simulink model "model"  (R2014a)
(part 2 of 2)

  _CN_199309340_110000_CN_171608231_110000/RConn2 -- T_171608231__RTP/LConn2 -- _CN_34853414_110000_CN_171608231_110000/LConn2
  _CN_199309340_110000_CN_171608231_110000/RConn3 -- T_171608231__RTP/LConn3 -- _CN_34853414_110000_CN_171608231_110000/LConn3 -- bus2/LConn1
  _CN_199309340_110000_CN_129377014_110000/RConn1 -- T_129377014__HE_Vuhred/LConn1 -- _CN_198773974_110000_CN_129377014_110000/LConn1 -- _CN_34853414_110000_CN_129377014_110000/LConn1
  _CN_199309340_110000_CN_129377014_110000/RConn2 -- T_129377014__HE_Vuhred/LConn2 -- _CN_198773974_110000_CN_129377014_110000/LConn2 -- _CN_34853414_110000_CN_129377014_110000/LConn2
  _CN_199309340_110000_CN_129377014_110000/RConn3 -- T_129377014__HE_Vuhred/LConn3 -- _CN_198773974_110000_CN_129377014_110000/LConn3 -- bus3/LConn1 -- _CN_34853414_110000_CN_129377014_110000/LConn3
  _CN_121547295_110000_CN_306834171_110000/LConn1 -- T_121547295_110000_HE_Mavčiče/LConn1 -- _CN_121547295_110000_CN_35041274_110000/LConn1 -- _CN_121547295_110000_CN_167068843_110000/LConn1
  _CN_121547295_110000_CN_306834171_110000/LConn2 -- T_121547295_110000_HE_Mavčiče/LConn2 -- _CN_121547295_110000_CN_35041274_110000/LConn2 -- _CN_121547295_110000_CN_167068843_110000/LConn2
  _CN_121547295_110000_CN_306834171_110000/LConn3 -- T_121547295_110000_HE_Mavčiče/LConn3 -- _CN_121547295_110000_CN_35041274_110000/LConn3 -- _CN_121547295_110000_CN_167068843_110000/LConn3 -- bus4/LConn1
  _CN_121547295_110000_CN_306834171_110000/RConn1 -- T_306834171__RTP_Labore/LConn1 -- _CN_306834171_110000_CN_306834179_110000/LConn1
  _CN_121547295_110000_CN_306834171_110000/RConn2 -- T_306834171__RTP_Labore/LConn2 -- _CN_306834171_110000_CN_306834179_110000/LConn2
  _CN_121547295_110000_CN_306834171_110000/RConn3 -- T_306834171__RTP_Labore/LConn3 -- _CN_306834171_110000_CN_306834179_110000/LConn3 -- bus5/LConn1
  _CN_121547295_110000_CN_35041274_110000/RConn1 -- T_35041274__RTP_Okroglo/RConn1 -- _CN_306834179_110000_CN_35041274_110000/LConn1 -- L_35041274/LConn1 -- _CN_167068843_110000_CN_35041274_110000/LConn1
  _CN_121547295_110000_CN_35041274_110000/RConn2 -- T_35041274__RTP_Okroglo/RConn2 -- _CN_306834179_110000_CN_35041274_110000/LConn2 -- L_35041274/LConn2 -- _CN_167068843_110000_CN_35041274_110000/LConn2
  _CN_121547295_110000_CN_35041274_110000/RConn3 -- T_35041274__RTP_Okroglo/RConn3 -- _CN_306834179_110000_CN_35041274_110000/LConn3 -- L_35041274/LConn3 -- bus6/LConn1 -- _CN_167068843_110000_CN_35041274_110000/LConn3
  _CN_121547295_110000_CN_167068843_110000/RConn1 -- T_167068843_220000;110000_RTP_Kleče/LConn1 -- _CN_167068843_110000_CN_198965564_110000/LConn1 -- 2x110_kV_TE_TOL___Črnuče___Kleče_CN_167068843_110000_CN_186330420_110000/LConn1 -- 2x110_kV_TE_TOL___Črnuče___Kleče_CN_167068843_110000_CN_35073279_110000/LConn1 -- _CN_167068843_110000_CN_138362793_110000/LConn1 -- _CN_199456347_110000_CN_167068843_110000/LConn1 -- _CN_199456348_110000_CN_167068843_110000/LConn1 -- _CN_199131958_110000_CN_167068843_110000/LConn1 -- _CN_167068843_110000_CN_306834196_110000/LConn1 -- _CN_167068843_110000_CN_35041274_110000/RConn1
  _CN_121547295_110000_CN_167068843_110000/RConn2 -- T_167068843_220000;110000_RTP_Kleče/LConn2 -- _CN_167068843_110000_CN_198965564_110000/LConn2 -- 2x110_kV_TE_TOL___Črnuče___Kleče_CN_167068843_110000_CN_186330420_110000/LConn2 -- 2x110_kV_TE_TOL___Črnuče___Kleče_CN_167068843_110000_CN_35073279_110000/LConn2 -- _CN_167068843_110000_CN_138362793_110000/LConn2 -- _CN_199456347_110000_CN_167068843_110000/LConn2 -- _CN_199456348_110000_CN_167068843_110000/LConn2 -- _CN_199131958_110000_CN_167068843_110000/LConn2 -- _CN_167068843_110000_CN_306834196_110000/LConn2 -- _CN_167068843_110000_CN_35041274_110000/RConn2
  _CN_121547295_110000_CN_167068843_110000/RConn3 -- T_167068843_220000;110000_RTP_Kleče/LConn3 -- _CN_167068843_110000_CN_198965564_110000/LConn3 -- 2x110_kV_TE_TOL___Črnuče___Kleče_CN_167068843_110000_CN_186330420_110000/LConn3 -- 2x110_kV_TE_TOL___Črnuče___Kleče_CN_167068843_110000_CN_35073279_110000/LConn3 -- _CN_167068843_110000_CN_138362793_110000/LConn3 -- bus7/LConn1 -- _CN_199456347_110000_CN_167068843_110000/LConn3 -- _CN_199456348_110000_CN_167068843_110000/LConn3 -- _CN_199131958_110000_CN_167068843_110000/LConn3 -- _CN_167068843_110000_CN_306834196_110000/LConn3 -- _CN_167068843_110000_CN_35041274_110000/RConn3
  _CN_34853414_110000_CN_171608231_110000/RConn1 -- T_34853414__RTP_Pekre/LConn1 -- _CN_34853414_110000_CN_129377014_110000/RConn1 -- _CN_34853414_110000_CN_113578863_110000/LConn1 -- _CN_34853414_110000_CN_171257375_110000/LConn1 -- _CN_34853414_110000_CN_171247394_110000/LConn1 -- 110kV_podzemni_kabel_RTP_Koroška_vrata_RTP_Pekre_CN_34853414_110000_CN_171242382_110000/LConn1 -- _CN_34853414_110000_CN_170856590_110000/LConn1
  _CN_34853414_110000_CN_171608231_110000/RConn2 -- T_34853414__RTP_Pekre/LConn2 -- _CN_34853414_110000_CN_129377014_110000/RConn2 -- _CN_34853414_110000_CN_113578863_110000/LConn2 -- _CN_34853414_110000_CN_171257375_110000/LConn2 -- _CN_34853414_110000_CN_171247394_110000/LConn2 -- 110kV_podzemni_kabel_RTP_Koroška_vrata_RTP_Pekre_CN_34853414_110000_CN_171242382_110000/LConn2 -- _CN_34853414_110000_CN_170856590_110000/LConn2
  _CN_34853414_110000_CN_171608231_110000/RConn3 -- T_34853414__RTP_Pekre/LConn3 -- _CN_34853414_110000_CN_129377014_110000/RConn3 -- bus8/LConn1 -- _CN_34853414_110000_CN_113578863_110000/LConn3 -- _CN_34853414_110000_CN_171257375_110000/LConn3 -- _CN_34853414_110000_CN_171247394_110000/LConn3 -- 110kV_podzemni_kabel_RTP_Koroška_vrata_RTP_Pekre_CN_34853414_110000_CN_171242382_110000/LConn3 -- _CN_34853414_110000_CN_170856590_110000/LConn3
  _CN_34853414_110000_CN_113578863_110000/RConn1 -- T_113578863__RTP_Maribor/RConn1 -- 110kV_RTP_Maribor_RTP_Lenart_CN_113578863_110000_CN_171246987_110000/LConn1 -- 110_kV_RTP_Maribor_RTP_Melje_CN_113578863_110000_CN_171242383_110000/LConn1 -- L_113578863/LConn1 -- 110kV_RTP_Maribor_RTP_Cirkovce_CN_113568896_110000_CN_113578863_110000/LConn1
  _CN_34853414_110000_CN_113578863_110000/RConn2 -- T_113578863__RTP_Maribor/RConn2 -- 110kV_RTP_Maribor_RTP_Lenart_CN_113578863_110000_CN_171246987_110000/LConn2 -- 110_kV_RTP_Maribor_RTP_Melje_CN_113578863_110000_CN_171242383_110000/LConn2 -- L_113578863/LConn2 -- 110kV_RTP_Maribor_RTP_Cirkovce_CN_113568896_110000_CN_113578863_110000/LConn2
  _CN_34853414_110000_CN_113578863_110000/RConn3 -- T_113578863__RTP_Maribor/RConn3 -- 110kV_RTP_Maribor_RTP_Lenart_CN_113578863_110000_CN_171246987_110000/LConn3 -- 110_kV_RTP_Maribor_RTP_Melje_CN_113578863_110000_CN_171242383_110000/LConn3 -- L_113578863/LConn3 -- bus9/LConn1 -- 110kV_RTP_Maribor_RTP_Cirkovce_CN_113568896_110000_CN_113578863_110000/LConn3
  T_171257375__RTP_Slovenska_BIstrica/LConn1 -- _CN_34853414_110000_CN_171257375_110000/RConn1
  T_171257375__RTP_Slovenska_BIstrica/LConn2 -- _CN_34853414_110000_CN_171257375_110000/RConn2
  _CN_34853414_110000_CN_171257375_110000/RConn3 -- T_171257375__RTP_Slovenska_BIstrica/LConn3 -- bus10/LConn1
  T_171247394__HE_Mariborski_otok/LConn1 -- _CN_34853414_110000_CN_171247394_110000/RConn1
  T_171247394__HE_Mariborski_otok/LConn2 -- _CN_34853414_110000_CN_171247394_110000/RConn2
  _CN_34853414_110000_CN_171247394_110000/RConn3 -- T_171247394__HE_Mariborski_otok/LConn3 -- bus11/LConn1
  110kV_podzemni_kabel_RTP_Koroška_vrata_RTP_Pekre_CN_34853414_110000_CN_171242382_110000/RConn1 -- T_171242382__RTP_Koroška_vrata/LConn1 -- 110kV_podvodni_kabel_RTP_Koroška_vrata__RTP_Melje_CN_171242382_110000_CN_171242383_110000/LConn1
  110kV_podzemni_kabel_RTP_Koroška_vrata_RTP_Pekre_CN_34853414_110000_CN_171242382_110000/RConn2 -- T_171242382__RTP_Koroška_vrata/LConn2 -- 110kV_podvodni_kabel_RTP_Koroška_vrata__RTP_Melje_CN_171242382_110000_CN_171242383_110000/LConn2
  110kV_podzemni_kabel_RTP_Koroška_vrata_RTP_Pekre_CN_34853414_110000_CN_171242382_110000/RConn3 -- T_171242382__RTP_Koroška_vrata/LConn3 -- 110kV_podvodni_kabel_RTP_Koroška_vrata__RTP_Melje_CN_171242382_110000_CN_171242383_110000/LConn3 -- bus12/LConn1
  T_170856590__RTP_Dobrava/LConn1 -- _CN_34853414_110000_CN_170856590_110000/RConn1
  T_170856590__RTP_Dobrava/LConn2 -- _CN_34853414_110000_CN_170856590_110000/RConn2
  _CN_34853414_110000_CN_170856590_110000/RConn3 -- T_170856590__RTP_Dobrava/LConn3 -- bus13/LConn1
  T_280821359__/LConn1 -- _CN_280821359_110000_CN_171277752_110000/LConn1
  T_280821359__/LConn2 -- _CN_280821359_110000_CN_171277752_110000/LConn2
  _CN_280821359_110000_CN_171277752_110000/LConn3 -- T_280821359__/LConn3 -- bus14/LConn1
  T_171277752__RTP_Slovenske_Konjice/LConn1 -- _CN_280821359_110000_CN_171277752_110000/RConn1
  T_171277752__RTP_Slovenske_Konjice/LConn2 -- _CN_280821359_110000_CN_171277752_110000/RConn2
  _CN_280821359_110000_CN_171277752_110000/RConn3 -- T_171277752__RTP_Slovenske_Konjice/LConn3 -- bus15/LConn1
  _CN_171047486_110000_CN_113568896_110000/LConn1 -- T_171047486__RTP_Kidričevo/LConn1 -- _CN_171047486_110000_CN_171223453_110000/LConn1 -- _CN_171047486_110000_CN_171127243_110000/LConn1
  _CN_171047486_110000_CN_113568896_110000/LConn2 -- T_171047486__RTP_Kidričevo/LConn2 -- _CN_171047486_110000_CN_171223453_110000/LConn2 -- _CN_171047486_110000_CN_171127243_110000/LConn2
  _CN_171047486_110000_CN_113568896_110000/LConn3 -- T_171047486__RTP_Kidričevo/LConn3 -- _CN_171047486_110000_CN_171223453_110000/LConn3 -- _CN_171047486_110000_CN_171127243_110000/LConn3 -- bus16/LConn1
  _CN_171047486_110000_CN_113568896_110000/RConn1 -- T_113568896__RTP_Cirkovce/LConn1 -- _CN_280821361_110000_CN_113568896_110000/LConn1 -- 110kV_RTP_Maribor_RTP_Cirkovce_CN_113568896_110000_CN_113578863_110000/RConn1 -- _CN_113568896_110000_CN_170978399_110000/LConn1
  _CN_171047486_110000_CN_113568896_110000/RConn2 -- T_113568896__RTP_Cirkovce/LConn2 -- _CN_280821361_110000_CN_113568896_110000/LConn2 -- 110kV_RTP_Maribor_RTP_Cirkovce_CN_113568896_110000_CN_113578863_110000/RConn2 -- _CN_113568896_110000_CN_170978399_110000/LConn2
  _CN_171047486_110000_CN_113568896_110000/RConn3 -- T_113568896__RTP_Cirkovce/LConn3 -- _CN_280821361_110000_CN_113568896_110000/LConn3 -- 110kV_RTP_Maribor_RTP_Cirkovce_CN_113568896_110000_CN_113578863_110000/RConn3 -- _CN_113568896_110000_CN_170978399_110000/LConn3 -- bus17/LConn1
  _CN_171047486_110000_CN_171223453_110000/RConn1 -- G_171223453_HE_Formin/RConn1 -- _CN_171229302_110000_CN_171223453_110000/LConn1 -- _CN_280821361_110000_CN_171223453_110000/LConn1
  _CN_171047486_110000_CN_171223453_110000/RConn2 -- G_171223453_HE_Formin/RConn2 -- _CN_171229302_110000_CN_171223453_110000/LConn2 -- _CN_280821361_110000_CN_171223453_110000/LConn2
  _CN_171047486_110000_CN_171223453_110000/RConn3 -- G_171223453_HE_Formin/RConn3 -- _CN_171229302_110000_CN_171223453_110000/LConn3 -- bus18/LConn1 -- _CN_280821361_110000_CN_171223453_110000/LConn3
  T_171127243__RTP_Ptuj/LConn1 -- _CN_171047486_110000_CN_171127243_110000/RConn1
  T_171127243__RTP_Ptuj/LConn2 -- _CN_171047486_110000_CN_171127243_110000/RConn2
  _CN_171047486_110000_CN_171127243_110000/RConn3 -- T_171127243__RTP_Ptuj/LConn3 -- bus19/LConn1
  T_198587974__RTP/LConn1 -- Podlog_Mozirje_CN_198587974_110000_CN_119244495_110000/LConn1
  T_198587974__RTP/LConn2 -- Podlog_Mozirje_CN_198587974_110000_CN_119244495_110000/LConn2
  Podlog_Mozirje_CN_198587974_110000_CN_119244495_110000/LConn3 -- T_198587974__RTP/LConn3 -- bus20/LConn1
  Podlog_Mozirje_CN_198587974_110000_CN_119244495_110000/RConn1 -- T_119244495__RTP_Podlog/RConn1 -- _CN_280821368_110000_CN_119244495_110000/LConn1 -- L_119244495/LConn1
  Podlog_Mozirje_CN_198587974_110000_CN_119244495_110000/RConn2 -- T_119244495__RTP_Podlog/RConn2 -- _CN_280821368_110000_CN_119244495_110000/LConn2 -- L_119244495/LConn2
  Podlog_Mozirje_CN_198587974_110000_CN_119244495_110000/RConn3 -- T_119244495__RTP_Podlog/RConn3 -- _CN_280821368_110000_CN_119244495_110000/LConn3 -- L_119244495/LConn3 -- bus21/LConn1
  T_199456336__RTP_Bršljin/LConn1 -- _CN_199456336_110000_CN_198740080_110000/LConn1
  T_199456336__RTP_Bršljin/LConn2 -- _CN_199456336_110000_CN_198740080_110000/LConn2
  _CN_199456336_110000_CN_198740080_110000/LConn3 -- T_199456336__RTP_Bršljin/LConn3 -- bus22/LConn1
  _CN_199456336_110000_CN_198740080_110000/RConn1 -- T_198740080_110000_RP_Hudo/LConn1 -- _CN_198740080_110000_CN_262103358_110000/LConn1 -- _CN_198740080_110000_CN_262103381_110000/LConn1
  _CN_199456336_110000_CN_198740080_110000/RConn2 -- T_198740080_110000_RP_Hudo/LConn2 -- _CN_198740080_110000_CN_262103358_110000/LConn2 -- _CN_198740080_110000_CN_262103381_110000/LConn2
  _CN_199456336_110000_CN_198740080_110000/RConn3 -- T_198740080_110000_RP_Hudo/LConn3 -- _CN_198740080_110000_CN_262103358_110000/LConn3 -- _CN_198740080_110000_CN_262103381_110000/LConn3 -- bus23/LConn1
  T_199456340_110000_RTP_Grosuplje/LConn1 -- _CN_199456340_110000_CN_138362793_110000/LConn1
  T_199456340_110000_RTP_Grosuplje/LConn2 -- _CN_199456340_110000_CN_138362793_110000/LConn2
  _CN_199456340_110000_CN_138362793_110000/LConn3 -- T_199456340_110000_RTP_Grosuplje/LConn3 -- bus24/LConn1
  _CN_199456340_110000_CN_138362793_110000/RConn1 -- T_138362793__RTP_Beričevo/RConn1 -- _CN_167068843_110000_CN_138362793_110000/RConn1 -- 2x110_kV_TE_TOL___Polje___Beričevo_CN_138362793_110000_CN_35073279_110000/LConn1 -- L_138362793/LConn1
  _CN_199456340_110000_CN_138362793_110000/RConn2 -- T_138362793__RTP_Beričevo/RConn2 -- _CN_167068843_110000_CN_138362793_110000/RConn2 -- 2x110_kV_TE_TOL___Polje___Beričevo_CN_138362793_110000_CN_35073279_110000/LConn2 -- L_138362793/LConn2
  _CN_199456340_110000_CN_138362793_110000/RConn3 -- T_138362793__RTP_Beričevo/RConn3 -- _CN_167068843_110000_CN_138362793_110000/RConn3 -- 2x110_kV_TE_TOL___Polje___Beričevo_CN_138362793_110000_CN_35073279_110000/LConn3 -- L_138362793/LConn3 -- bus25/LConn1
  T_199456341__RTP_Kamnik/LConn1 -- Domžale___Kamnik_CN_199456341_110000_CN_198965564_110000/LConn1
  T_199456341__RTP_Kamnik/LConn2 -- Domžale___Kamnik_CN_199456341_110000_CN_198965564_110000/LConn2
  Domžale___Kamnik_CN_199456341_110000_CN_198965564_110000/LConn3 -- T_199456341__RTP_Kamnik/LConn3 -- bus26/LConn1
  Domžale___Kamnik_CN_199456341_110000_CN_198965564_110000/RConn1 -- T_198965564__RTP_Domžale/LConn1 -- _CN_167068843_110000_CN_198965564_110000/RConn1
  Domžale___Kamnik_CN_199456341_110000_CN_198965564_110000/RConn2 -- T_198965564__RTP_Domžale/LConn2 -- _CN_167068843_110000_CN_198965564_110000/RConn2
  Domžale___Kamnik_CN_199456341_110000_CN_198965564_110000/RConn3 -- T_198965564__RTP_Domžale/LConn3 -- _CN_167068843_110000_CN_198965564_110000/RConn3 -- bus27/LConn1
  T_199456345__RTP_Potoška_vas/LConn1 -- _CN_199456345_110000_CN_286599451_110000/LConn1
  T_199456345__RTP_Potoška_vas/LConn2 -- _CN_199456345_110000_CN_286599451_110000/LConn2
  _CN_199456345_110000_CN_286599451_110000/LConn3 -- T_199456345__RTP_Potoška_vas/LConn3 -- bus28/LConn1
  T_286599451__RTP_Trbovlje/LConn1 -- _CN_199456345_110000_CN_286599451_110000/RConn1
  T_286599451__RTP_Trbovlje/LConn2 -- _CN_199456345_110000_CN_286599451_110000/RConn2
  _CN_199456345_110000_CN_286599451_110000/RConn3 -- T_286599451__RTP_Trbovlje/LConn3 -- bus29/LConn1
  T_199456347__RTP_Vič/LConn1 -- _CN_199456347_110000_CN_167068843_110000/RConn1
  T_199456347__RTP_Vič/LConn2 -- _CN_199456347_110000_CN_167068843_110000/RConn2
  _CN_199456347_110000_CN_167068843_110000/RConn3 -- T_199456347__RTP_Vič/LConn3 -- bus30/LConn1
  T_199456348__RTP_Šiška/LConn1 -- _CN_199456348_110000_CN_167068843_110000/RConn1
  T_199456348__RTP_Šiška/LConn2 -- _CN_199456348_110000_CN_167068843_110000/RConn2
  _CN_199456348_110000_CN_167068843_110000/RConn3 -- T_199456348__RTP_Šiška/LConn3 -- bus31/LConn1
  T_198740079__/LConn1 -- _CN_198740079_110000_CN_262103381_110000/LConn1
  T_198740079__/LConn2 -- _CN_198740079_110000_CN_262103381_110000/LConn2
  _CN_198740079_110000_CN_262103381_110000/LConn3 -- T_198740079__/LConn3 -- bus32/LConn1
  _CN_198740079_110000_CN_262103381_110000/RConn1 -- T_262103381__/LConn1 -- _CN_198740080_110000_CN_262103381_110000/RConn1
  _CN_198740079_110000_CN_262103381_110000/RConn2 -- T_262103381__/LConn2 -- _CN_198740080_110000_CN_262103381_110000/RConn2
  _CN_198740079_110000_CN_262103381_110000/RConn3 -- T_262103381__/LConn3 -- _CN_198740080_110000_CN_262103381_110000/RConn3 -- bus33/LConn1
  _CN_306794096_110000_CN_370156011_110000/LConn1 -- T_306794096_110000_HE_Plave/LConn1 -- _CN_306794096_110000_CN_369889751_110000/LConn1
  _CN_306794096_110000_CN_370156011_110000/LConn2 -- T_306794096_110000_HE_Plave/LConn2 -- _CN_306794096_110000_CN_369889751_110000/LConn2
  _CN_306794096_110000_CN_370156011_110000/LConn3 -- T_306794096_110000_HE_Plave/LConn3 -- _CN_306794096_110000_CN_369889751_110000/LConn3 -- bus34/LConn1
  T_370156011__RTP_Anhovo/LConn1 -- _CN_306794096_110000_CN_370156011_110000/RConn1
  T_370156011__RTP_Anhovo/LConn2 -- _CN_306794096_110000_CN_370156011_110000/RConn2
  _CN_306794096_110000_CN_370156011_110000/RConn3 -- T_370156011__RTP_Anhovo/LConn3 -- bus35/LConn1
  _CN_306794096_110000_CN_369889751_110000/RConn1 -- G_369889751_ČHE_Avče/RConn1 -- _CN_306692448_110000_CN_369889751_110000/LConn1
  _CN_306794096_110000_CN_369889751_110000/RConn2 -- G_369889751_ČHE_Avče/RConn2 -- _CN_306692448_110000_CN_369889751_110000/LConn2
  _CN_306794096_110000_CN_369889751_110000/RConn3 -- G_369889751_ČHE_Avče/RConn3 -- _CN_306692448_110000_CN_369889751_110000/LConn3 -- bus36/LConn1
  _CN_280821361_110000_CN_280821367_110000/LConn1 -- T_280821361__/LConn1 -- _CN_280821361_110000_CN_171223453_110000/RConn1 -- _CN_280821361_110000_CN_113568896_110000/RConn1
  _CN_280821361_110000_CN_280821367_110000/LConn2 -- T_280821361__/LConn2 -- _CN_280821361_110000_CN_171223453_110000/RConn2 -- _CN_280821361_110000_CN_113568896_110000/RConn2
  _CN_280821361_110000_CN_280821367_110000/LConn3 -- T_280821361__/LConn3 -- _CN_280821361_110000_CN_171223453_110000/RConn3 -- _CN_280821361_110000_CN_113568896_110000/RConn3 -- bus37/LConn1
  T_280821367__/LConn1 -- _CN_280821361_110000_CN_280821367_110000/RConn1
  T_280821367__/LConn2 -- _CN_280821361_110000_CN_280821367_110000/RConn2
  _CN_280821361_110000_CN_280821367_110000/RConn3 -- T_280821367__/LConn3 -- bus38/LConn1
  _CN_199131958_110000_CN_167068843_110000/RConn1 -- T_199131958__RTP_Logatec/LConn1 -- _CN_199131958_110000_CN_199131955_110000/LConn1
  _CN_199131958_110000_CN_167068843_110000/RConn2 -- T_199131958__RTP_Logatec/LConn2 -- _CN_199131958_110000_CN_199131955_110000/LConn2
  _CN_199131958_110000_CN_167068843_110000/RConn3 -- T_199131958__RTP_Logatec/LConn3 -- _CN_199131958_110000_CN_199131955_110000/LConn3 -- bus39/LConn1
  T_199131955__RTP_Vrhnika/LConn1 -- _CN_199131958_110000_CN_199131955_110000/RConn1
  T_199131955__RTP_Vrhnika/LConn2 -- _CN_199131958_110000_CN_199131955_110000/RConn2
  _CN_199131958_110000_CN_199131955_110000/RConn3 -- T_199131955__RTP_Vrhnika/LConn3 -- bus40/LConn1
  T_172406389__RTP_Radenci/LConn1 -- RTP_Murska_Sobota_RTP_Radenci_CN_172406389_110000_CN_172405235_110000/LConn1
  T_172406389__RTP_Radenci/LConn2 -- RTP_Murska_Sobota_RTP_Radenci_CN_172406389_110000_CN_172405235_110000/LConn2
  RTP_Murska_Sobota_RTP_Radenci_CN_172406389_110000_CN_172405235_110000/LConn3 -- T_172406389__RTP_Radenci/LConn3 -- bus41/LConn1
  RTP_Murska_Sobota_RTP_Radenci_CN_172406389_110000_CN_172405235_110000/RConn1 -- T_172405235__RTP_Murska_Sobota/LConn1 -- RTP_Ljutomer_RTP_Murska_Sobota_CN_171229302_110000_CN_172405235_110000/LConn1
  RTP_Murska_Sobota_RTP_Radenci_CN_172406389_110000_CN_172405235_110000/RConn2 -- T_172405235__RTP_Murska_Sobota/LConn2 -- RTP_Ljutomer_RTP_Murska_Sobota_CN_171229302_110000_CN_172405235_110000/LConn2
  RTP_Murska_Sobota_RTP_Radenci_CN_172406389_110000_CN_172405235_110000/RConn3 -- T_172405235__RTP_Murska_Sobota/LConn3 -- RTP_Ljutomer_RTP_Murska_Sobota_CN_171229302_110000_CN_172405235_110000/LConn3 -- bus42/LConn1
  _CN_171229302_110000_CN_200118427_110000/LConn1 -- T_171229302__RTP_Ljutomer/LConn1 -- RTP_Ljutomer_RTP_Murska_Sobota_CN_171229302_110000_CN_172405235_110000/RConn1 -- _CN_171229302_110000_CN_171227992_110000/LConn1 -- _CN_171229302_110000_CN_171223453_110000/RConn1
  _CN_171229302_110000_CN_200118427_110000/LConn2 -- T_171229302__RTP_Ljutomer/LConn2 -- RTP_Ljutomer_RTP_Murska_Sobota_CN_171229302_110000_CN_172405235_110000/RConn2 -- _CN_171229302_110000_CN_171227992_110000/LConn2 -- _CN_171229302_110000_CN_171223453_110000/RConn2
  _CN_171229302_110000_CN_200118427_110000/LConn3 -- T_171229302__RTP_Ljutomer/LConn3 -- RTP_Ljutomer_RTP_Murska_Sobota_CN_171229302_110000_CN_172405235_110000/RConn3 -- _CN_171229302_110000_CN_171227992_110000/LConn3 -- _CN_171229302_110000_CN_171223453_110000/RConn3 -- bus43/LConn1
  T_200118427__/LConn1 -- _CN_171229302_110000_CN_200118427_110000/RConn1
  T_200118427__/LConn2 -- _CN_171229302_110000_CN_200118427_110000/RConn2
  _CN_171229302_110000_CN_200118427_110000/RConn3 -- T_200118427__/LConn3 -- bus44/LConn1
  T_171227992__RTP_Ormož/LConn1 -- _CN_171229302_110000_CN_171227992_110000/RConn1
  T_171227992__RTP_Ormož/LConn2 -- _CN_171229302_110000_CN_171227992_110000/RConn2
  _CN_171229302_110000_CN_171227992_110000/RConn3 -- T_171227992__RTP_Ormož/LConn3 -- bus45/LConn1
  T_280821368__/LConn1 -- _CN_280821368_110000_CN_119244495_110000/RConn1
  T_280821368__/LConn2 -- _CN_280821368_110000_CN_119244495_110000/RConn2
  _CN_280821368_110000_CN_119244495_110000/RConn3 -- T_280821368__/LConn3 -- bus46/LConn1
  G_170978399_HE_Zlatoličje/RConn1 -- _CN_113568896_110000_CN_170978399_110000/RConn1
  G_170978399_HE_Zlatoličje/RConn2 -- _CN_113568896_110000_CN_170978399_110000/RConn2
  _CN_113568896_110000_CN_170978399_110000/RConn3 -- G_170978399_HE_Zlatoličje/RConn3 -- bus47/LConn1
  T_262103358__/LConn1 -- _CN_198740080_110000_CN_262103358_110000/RConn1
  T_262103358__/LConn2 -- _CN_198740080_110000_CN_262103358_110000/RConn2
  _CN_198740080_110000_CN_262103358_110000/RConn3 -- T_262103358__/LConn3 -- bus48/LConn1
  DV_Krapina___Straža_CN_159593130_110000_CN_208625989_110000/LConn1 -- T_159593130__TS_Straža/LConn1 -- DV_Ivanec___Straža_CN_159593130_110000_CN_99634141_110000/LConn1
  DV_Krapina___Straža_CN_159593130_110000_CN_208625989_110000/LConn2 -- T_159593130__TS_Straža/LConn2 -- DV_Ivanec___Straža_CN_159593130_110000_CN_99634141_110000/LConn2
  DV_Krapina___Straža_CN_159593130_110000_CN_208625989_110000/LConn3 -- T_159593130__TS_Straža/LConn3 -- DV_Ivanec___Straža_CN_159593130_110000_CN_99634141_110000/LConn3 -- bus49/LConn1
  T_208625989__/LConn1 -- DV_Krapina___Straža_CN_159593130_110000_CN_208625989_110000/RConn1
  T_208625989__/LConn2 -- DV_Krapina___Straža_CN_159593130_110000_CN_208625989_110000/RConn2
  DV_Krapina___Straža_CN_159593130_110000_CN_208625989_110000/RConn3 -- T_208625989__/LConn3 -- bus50/LConn1
  T_99634141__TS_Ivanec/LConn1 -- DV_Ivanec___Straža_CN_159593130_110000_CN_99634141_110000/RConn1
  T_99634141__TS_Ivanec/LConn2 -- DV_Ivanec___Straža_CN_159593130_110000_CN_99634141_110000/RConn2
  DV_Ivanec___Straža_CN_159593130_110000_CN_99634141_110000/RConn3 -- T_99634141__TS_Ivanec/LConn3 -- bus51/LConn1
  T_306834196__RTP_Škofja_Loka/LConn1 -- _CN_167068843_110000_CN_306834196_110000/RConn1
  T_306834196__RTP_Škofja_Loka/LConn2 -- _CN_167068843_110000_CN_306834196_110000/RConn2
  _CN_167068843_110000_CN_306834196_110000/RConn3 -- T_306834196__RTP_Škofja_Loka/LConn3 -- bus52/LConn1
  T_186330420__RTP_Črnuče/LConn1 -- 2x110_kV_TE_TOL___Črnuče___Kleče_CN_167068843_110000_CN_186330420_110000/RConn1
  T_186330420__RTP_Črnuče/LConn2 -- 2x110_kV_TE_TOL___Črnuče___Kleče_CN_167068843_110000_CN_186330420_110000/RConn2
  2x110_kV_TE_TOL___Črnuče___Kleče_CN_167068843_110000_CN_186330420_110000/RConn3 -- T_186330420__RTP_Črnuče/LConn3 -- bus53/LConn1
  2x110_kV_TE_TOL___Črnuče___Kleče_CN_167068843_110000_CN_35073279_110000/RConn1 -- G_35073279_Termoelektrarna_Toplarna_Ljubljana/RConn1 -- 2x110_kV_TE_TOL___Polje___Beričevo_CN_138362793_110000_CN_35073279_110000/RConn1 -- 110_kV_TE_TOL___Polje_CN_138362817_110000_CN_35073279_110000/LConn1
  2x110_kV_TE_TOL___Črnuče___Kleče_CN_167068843_110000_CN_35073279_110000/RConn2 -- G_35073279_Termoelektrarna_Toplarna_Ljubljana/RConn2 -- 2x110_kV_TE_TOL___Polje___Beričevo_CN_138362793_110000_CN_35073279_110000/RConn2 -- 110_kV_TE_TOL___Polje_CN_138362817_110000_CN_35073279_110000/LConn2
  2x110_kV_TE_TOL___Črnuče___Kleče_CN_167068843_110000_CN_35073279_110000/RConn3 -- G_35073279_Termoelektrarna_Toplarna_Ljubljana/RConn3 -- 2x110_kV_TE_TOL___Polje___Beričevo_CN_138362793_110000_CN_35073279_110000/RConn3 -- 110_kV_TE_TOL___Polje_CN_138362817_110000_CN_35073279_110000/LConn3 -- bus54/LConn1
  T_376534710__RTP/LConn1 -- Ajdovščina___Divača_CN_376534710_110000_CN_96747435_110000/LConn1
  T_376534710__RTP/LConn2 -- Ajdovščina___Divača_CN_376534710_110000_CN_96747435_110000/LConn2
  Ajdovščina___Divača_CN_376534710_110000_CN_96747435_110000/LConn3 -- T_376534710__RTP/LConn3 -- bus55/LConn1
  Ajdovščina___Divača_CN_376534710_110000_CN_96747435_110000/RConn1 -- T_96747435_400000;220000;110000_RTP_Divača/RConn1 -- _CN_199389074_110000_CN_96747435_110000/LConn1 -- L_96747435/LConn1 -- _CN_199131954_110000_CN_96747435_110000/LConn1 -- Divača___Sežana_CN_208270146_110000_CN_96747435_110000/LConn1
  Ajdovščina___Divača_CN_376534710_110000_CN_96747435_110000/RConn2 -- T_96747435_400000;220000;110000_RTP_Divača/RConn2 -- _CN_199389074_110000_CN_96747435_110000/LConn2 -- L_96747435/LConn2 -- _CN_199131954_110000_CN_96747435_110000/LConn2 -- Divača___Sežana_CN_208270146_110000_CN_96747435_110000/LConn2
  Ajdovščina___Divača_CN_376534710_110000_CN_96747435_110000/RConn3 -- T_96747435_400000;220000;110000_RTP_Divača/RConn3 -- _CN_199389074_110000_CN_96747435_110000/LConn3 -- L_96747435/LConn3 -- bus56/LConn1 -- _CN_199131954_110000_CN_96747435_110000/LConn3 -- Divača___Sežana_CN_208270146_110000_CN_96747435_110000/LConn3
  T_132468928_110000_Kraftwerk_Koralpe/LConn1 -- Lavamünd___Koralpe_CN_132468928_110000_CN_98291700_110000/LConn1
  T_132468928_110000_Kraftwerk_Koralpe/LConn2 -- Lavamünd___Koralpe_CN_132468928_110000_CN_98291700_110000/LConn2
  Lavamünd___Koralpe_CN_132468928_110000_CN_98291700_110000/LConn3 -- T_132468928_110000_Kraftwerk_Koralpe/LConn3 -- bus57/LConn1
  G_98291700_Kraftwerk_Lavamünd/RConn1 -- Lavamünd___Koralpe_CN_132468928_110000_CN_98291700_110000/RConn1
  G_98291700_Kraftwerk_Lavamünd/RConn2 -- Lavamünd___Koralpe_CN_132468928_110000_CN_98291700_110000/RConn2
  Lavamünd___Koralpe_CN_132468928_110000_CN_98291700_110000/RConn3 -- G_98291700_Kraftwerk_Lavamünd/RConn3 -- bus58/LConn1
  T_161693379__RTP/LConn1 -- _CN_161693379_110000_CN_198773972_110000/LConn1
  T_161693379__RTP/LConn2 -- _CN_161693379_110000_CN_198773972_110000/LConn2
  _CN_161693379_110000_CN_198773972_110000/LConn3 -- T_161693379__RTP/LConn3 -- bus59/LConn1
  _CN_161693379_110000_CN_198773972_110000/RConn1 -- T_198773972__/LConn1 -- _CN_198773972_110000_CN_198773974_110000/LConn1
  _CN_161693379_110000_CN_198773972_110000/RConn2 -- T_198773972__/LConn2 -- _CN_198773972_110000_CN_198773974_110000/LConn2
  _CN_161693379_110000_CN_198773972_110000/RConn3 -- T_198773972__/LConn3 -- _CN_198773972_110000_CN_198773974_110000/LConn3 -- bus60/LConn1
  T_128572102__TS_Matulji/LConn1 -- _CN_128572102_110000_CN_276296152_110000/LConn1
  T_128572102__TS_Matulji/LConn2 -- _CN_128572102_110000_CN_276296152_110000/LConn2
  _CN_128572102_110000_CN_276296152_110000/LConn3 -- T_128572102__TS_Matulji/LConn3 -- bus61/LConn1
  T_276296152__Ilirska_Bistrica/LConn1 -- _CN_128572102_110000_CN_276296152_110000/RConn1
  T_276296152__Ilirska_Bistrica/LConn2 -- _CN_128572102_110000_CN_276296152_110000/RConn2
  _CN_128572102_110000_CN_276296152_110000/RConn3 -- T_276296152__Ilirska_Bistrica/LConn3 -- bus62/LConn1
  _CN_198773972_110000_CN_198773974_110000/RConn1 -- T_198773974__RTP_Vuzenica/LConn1 -- _CN_198773974_110000_CN_129377014_110000/RConn1
  _CN_198773972_110000_CN_198773974_110000/RConn2 -- T_198773974__RTP_Vuzenica/LConn2 -- _CN_198773974_110000_CN_129377014_110000/RConn2
  _CN_198773972_110000_CN_198773974_110000/RConn3 -- T_198773974__RTP_Vuzenica/LConn3 -- _CN_198773974_110000_CN_129377014_110000/RConn3 -- bus63/LConn1
  _CN_306834171_110000_CN_306834179_110000/RConn1 -- T_306834179__RTP_Primskovo/LConn1 -- _CN_306834179_110000_CN_35041274_110000/RConn1
  _CN_306834171_110000_CN_306834179_110000/RConn2 -- T_306834179__RTP_Primskovo/LConn2 -- _CN_306834179_110000_CN_35041274_110000/RConn2
  _CN_306834171_110000_CN_306834179_110000/RConn3 -- T_306834179__RTP_Primskovo/LConn3 -- _CN_306834179_110000_CN_35041274_110000/RConn3 -- bus64/LConn1
  T_242310951_110000_RTP_Postojna/LConn1 -- _CN_242310951_110000_CN_199389074_110000/LConn1
  T_242310951_110000_RTP_Postojna/LConn2 -- _CN_242310951_110000_CN_199389074_110000/LConn2
  _CN_242310951_110000_CN_199389074_110000/LConn3 -- T_242310951_110000_RTP_Postojna/LConn3 -- bus65/LConn1
  _CN_242310951_110000_CN_199389074_110000/RConn1 -- T_199389074_110000_RTP_Pivka/LConn1 -- _CN_199389074_110000_CN_96747435_110000/RConn1
  _CN_242310951_110000_CN_199389074_110000/RConn2 -- T_199389074_110000_RTP_Pivka/LConn2 -- _CN_199389074_110000_CN_96747435_110000/RConn2
  _CN_242310951_110000_CN_199389074_110000/RConn3 -- T_199389074_110000_RTP_Pivka/LConn3 -- _CN_199389074_110000_CN_96747435_110000/RConn3 -- bus66/LConn1
  _CN_199131954_110000_CN_123454320_110000/LConn1 -- T_199131954__RTP_Koper/LConn1 -- _CN_199131954_110000_CN_96747435_110000/RConn1
  _CN_199131954_110000_CN_123454320_110000/LConn2 -- T_199131954__RTP_Koper/LConn2 -- _CN_199131954_110000_CN_96747435_110000/RConn2
  _CN_199131954_110000_CN_123454320_110000/LConn3 -- T_199131954__RTP_Koper/LConn3 -- _CN_199131954_110000_CN_96747435_110000/RConn3 -- bus67/LConn1
  T_123454320__TS_Buje/LConn1 -- _CN_199131954_110000_CN_123454320_110000/RConn1
  T_123454320__TS_Buje/LConn2 -- _CN_199131954_110000_CN_123454320_110000/RConn2
  _CN_199131954_110000_CN_123454320_110000/RConn3 -- T_123454320__TS_Buje/LConn3 -- bus68/LConn1
  Sežana___Vrtojba_CN_208270146_110000_CN_306692456_110000/LConn1 -- T_208270146__RTP/LConn1 -- Divača___Sežana_CN_208270146_110000_CN_96747435_110000/RConn1 -- Sežana___Vrtojba_CN_208270146_110000_CN_306692448_110000/LConn1
  Sežana___Vrtojba_CN_208270146_110000_CN_306692456_110000/LConn2 -- T_208270146__RTP/LConn2 -- Divača___Sežana_CN_208270146_110000_CN_96747435_110000/RConn2 -- Sežana___Vrtojba_CN_208270146_110000_CN_306692448_110000/LConn2
  Sežana___Vrtojba_CN_208270146_110000_CN_306692456_110000/LConn3 -- T_208270146__RTP/LConn3 -- Divača___Sežana_CN_208270146_110000_CN_96747435_110000/RConn3 -- bus69/LConn1 -- Sežana___Vrtojba_CN_208270146_110000_CN_306692448_110000/LConn3
  T_306692456_110000_RTP_Vrtojba/LConn1 -- Sežana___Vrtojba_CN_208270146_110000_CN_306692456_110000/RConn1
  T_306692456_110000_RTP_Vrtojba/LConn2 -- Sežana___Vrtojba_CN_208270146_110000_CN_306692456_110000/RConn2
  Sežana___Vrtojba_CN_208270146_110000_CN_306692456_110000/RConn3 -- T_306692456_110000_RTP_Vrtojba/LConn3 -- bus70/LConn1
  Sežana___Vrtojba_CN_208270146_110000_CN_306692448_110000/RConn1 -- T_306692448_110000_RTP_Nova_Gorica/LConn1 -- _CN_306692448_110000_CN_369889747_110000/LConn1 -- _CN_306692448_110000_CN_369889751_110000/RConn1
  Sežana___Vrtojba_CN_208270146_110000_CN_306692448_110000/RConn2 -- T_306692448_110000_RTP_Nova_Gorica/LConn2 -- _CN_306692448_110000_CN_369889747_110000/LConn2 -- _CN_306692448_110000_CN_369889751_110000/RConn2
  Sežana___Vrtojba_CN_208270146_110000_CN_306692448_110000/RConn3 -- T_306692448_110000_RTP_Nova_Gorica/LConn3 -- _CN_306692448_110000_CN_369889747_110000/LConn3 -- _CN_306692448_110000_CN_369889751_110000/RConn3 -- bus71/LConn1
  T_369889747_110000_RTP_Tolmin/LConn1 -- _CN_306692448_110000_CN_369889747_110000/RConn1
  T_369889747_110000_RTP_Tolmin/LConn2 -- _CN_306692448_110000_CN_369889747_110000/RConn2
  _CN_306692448_110000_CN_369889747_110000/RConn3 -- T_369889747_110000_RTP_Tolmin/LConn3 -- bus72/LConn1
  T_171246987__RTP_Lenart/LConn1 -- 110kV_RTP_Maribor_RTP_Lenart_CN_113578863_110000_CN_171246987_110000/RConn1
  T_171246987__RTP_Lenart/LConn2 -- 110kV_RTP_Maribor_RTP_Lenart_CN_113578863_110000_CN_171246987_110000/RConn2
  110kV_RTP_Maribor_RTP_Lenart_CN_113578863_110000_CN_171246987_110000/RConn3 -- T_171246987__RTP_Lenart/LConn3 -- bus73/LConn1
  110_kV_RTP_Maribor_RTP_Melje_CN_113578863_110000_CN_171242383_110000/RConn1 -- T_171242383__RTP_Melje/LConn1 -- 110kV_podvodni_kabel_RTP_Koroška_vrata__RTP_Melje_CN_171242382_110000_CN_171242383_110000/RConn1
  110_kV_RTP_Maribor_RTP_Melje_CN_113578863_110000_CN_171242383_110000/RConn2 -- T_171242383__RTP_Melje/LConn2 -- 110kV_podvodni_kabel_RTP_Koroška_vrata__RTP_Melje_CN_171242382_110000_CN_171242383_110000/RConn2
  110_kV_RTP_Maribor_RTP_Melje_CN_113578863_110000_CN_171242383_110000/RConn3 -- T_171242383__RTP_Melje/LConn3 -- 110kV_podvodni_kabel_RTP_Koroška_vrata__RTP_Melje_CN_171242382_110000_CN_171242383_110000/RConn3 -- bus74/LConn1
  T_138362817__RTP_Polje/LConn1 -- 110_kV_TE_TOL___Polje_CN_138362817_110000_CN_35073279_110000/RConn1
  T_138362817__RTP_Polje/LConn2 -- 110_kV_TE_TOL___Polje_CN_138362817_110000_CN_35073279_110000/RConn2
  110_kV_TE_TOL___Polje_CN_138362817_110000_CN_35073279_110000/RConn3 -- T_138362817__RTP_Polje/LConn3 -- bus75/LConn1
  _CN_105894370_400000_CN_89819245_400000/LConn1 -- T_105894370__RTP_Krško/LConn1 -- _CN_105894370_400000_CN_138362793_400000/LConn1 -- 400_kV_Mihovci_RTP_Krško_CN_105894370_400000_CN_119244495_400000/LConn1 -- 400_kV_Mihovci_RTP_Krško_CN_105894370_400000_CN_113578863_400000/LConn1
  _CN_105894370_400000_CN_89819245_400000/LConn2 -- T_105894370__RTP_Krško/LConn2 -- _CN_105894370_400000_CN_138362793_400000/LConn2 -- 400_kV_Mihovci_RTP_Krško_CN_105894370_400000_CN_119244495_400000/LConn2 -- 400_kV_Mihovci_RTP_Krško_CN_105894370_400000_CN_113578863_400000/LConn2
  _CN_105894370_400000_CN_89819245_400000/LConn3 -- T_105894370__RTP_Krško/LConn3 -- _CN_105894370_400000_CN_138362793_400000/LConn3 -- 400_kV_Mihovci_RTP_Krško_CN_105894370_400000_CN_119244495_400000/LConn3 -- 400_kV_Mihovci_RTP_Krško_CN_105894370_400000_CN_113578863_400000/LConn3 -- bus76/LConn1
  G_89819245_Nuklearna_elektrarna_Krško/RConn1 -- _CN_105894370_400000_CN_89819245_400000/RConn1
  G_89819245_Nuklearna_elektrarna_Krško/RConn2 -- _CN_105894370_400000_CN_89819245_400000/RConn2
  _CN_105894370_400000_CN_89819245_400000/RConn3 -- G_89819245_Nuklearna_elektrarna_Krško/RConn3 -- bus77/LConn1
  _CN_105894370_400000_CN_138362793_400000/RConn1 -- T_138362793__RTP_Beričevo/LConn1 -- 400_kV_RTP_Beričevo_RTP_Podlog_CN_138362793_400000_CN_119244495_400000/LConn1 -- 400_kV_RTP_Beričevo_RTP_Divača_CN_138362793_400000_CN_96747435_400000/LConn1 -- 400_kV_RTP_Beričevo_RTP_Okroglo_CN_138362793_400000_CN_35041274_400000/LConn1
  _CN_105894370_400000_CN_138362793_400000/RConn2 -- T_138362793__RTP_Beričevo/LConn2 -- 400_kV_RTP_Beričevo_RTP_Podlog_CN_138362793_400000_CN_119244495_400000/LConn2 -- 400_kV_RTP_Beričevo_RTP_Divača_CN_138362793_400000_CN_96747435_400000/LConn2 -- 400_kV_RTP_Beričevo_RTP_Okroglo_CN_138362793_400000_CN_35041274_400000/LConn2
  _CN_105894370_400000_CN_138362793_400000/RConn3 -- T_138362793__RTP_Beričevo/LConn3 -- 400_kV_RTP_Beričevo_RTP_Podlog_CN_138362793_400000_CN_119244495_400000/LConn3 -- 400_kV_RTP_Beričevo_RTP_Divača_CN_138362793_400000_CN_96747435_400000/LConn3 -- bus78/LConn1 -- 400_kV_RTP_Beričevo_RTP_Okroglo_CN_138362793_400000_CN_35041274_400000/LConn3
  400_kV_Mihovci_RTP_Krško_CN_105894370_400000_CN_119244495_400000/RConn1 -- T_119244495__RTP_Podlog/LConn1 -- 400_kV_RTP_Beričevo_RTP_Podlog_CN_138362793_400000_CN_119244495_400000/RConn1 -- 400_kV_RTP_Šoštanj_RTP_Podlog_CN_119244495_400000_CN_119239942_400000/LConn1
  400_kV_Mihovci_RTP_Krško_CN_105894370_400000_CN_119244495_400000/RConn2 -- T_119244495__RTP_Podlog/LConn2 -- 400_kV_RTP_Beričevo_RTP_Podlog_CN_138362793_400000_CN_119244495_400000/RConn2 -- 400_kV_RTP_Šoštanj_RTP_Podlog_CN_119244495_400000_CN_119239942_400000/LConn2
  400_kV_Mihovci_RTP_Krško_CN_105894370_400000_CN_119244495_400000/RConn3 -- T_119244495__RTP_Podlog/LConn3 -- 400_kV_RTP_Beričevo_RTP_Podlog_CN_138362793_400000_CN_119244495_400000/RConn3 -- 400_kV_RTP_Šoštanj_RTP_Podlog_CN_119244495_400000_CN_119239942_400000/LConn3 -- bus79/LConn1
  T_113578863__RTP_Maribor/LConn1 -- 400_kV_Mihovci_RTP_Krško_CN_105894370_400000_CN_113578863_400000/RConn1
  T_113578863__RTP_Maribor/LConn2 -- 400_kV_Mihovci_RTP_Krško_CN_105894370_400000_CN_113578863_400000/RConn2
  400_kV_Mihovci_RTP_Krško_CN_105894370_400000_CN_113578863_400000/RConn3 -- T_113578863__RTP_Maribor/LConn3 -- bus80/LConn1
  T_35041274__RTP_Okroglo/LConn1 -- 400_kV_RTP_Beričevo_RTP_Okroglo_CN_138362793_400000_CN_35041274_400000/RConn1
  T_35041274__RTP_Okroglo/LConn2 -- 400_kV_RTP_Beričevo_RTP_Okroglo_CN_138362793_400000_CN_35041274_400000/RConn2
  400_kV_RTP_Beričevo_RTP_Okroglo_CN_138362793_400000_CN_35041274_400000/RConn3 -- T_35041274__RTP_Okroglo/LConn3 -- bus81/LConn1
  400_kV_RTP_Beričevo_RTP_Divača_CN_138362793_400000_CN_96747435_400000/RConn1 -- T_96747435_400000;220000;110000_RTP_Divača/LConn1 -- DV_Melina___Divača_CN_96747435_400000_CN_89817617_400000/LConn1
  400_kV_RTP_Beričevo_RTP_Divača_CN_138362793_400000_CN_96747435_400000/RConn2 -- T_96747435_400000;220000;110000_RTP_Divača/LConn2 -- DV_Melina___Divača_CN_96747435_400000_CN_89817617_400000/LConn2
  400_kV_RTP_Beričevo_RTP_Divača_CN_138362793_400000_CN_96747435_400000/RConn3 -- T_96747435_400000;220000;110000_RTP_Divača/LConn3 -- DV_Melina___Divača_CN_96747435_400000_CN_89817617_400000/LConn3 -- bus82/LConn1
  DV_Melina___Divača_CN_96747435_400000_CN_89817617_400000/RConn1 -- T_89817617_400000_TS_Melina/LConn1 -- DV_Tumbri___Melina_CN_89817617_400000_CN_89818719_400000/LConn1
  DV_Melina___Divača_CN_96747435_400000_CN_89817617_400000/RConn2 -- T_89817617_400000_TS_Melina/LConn2 -- DV_Tumbri___Melina_CN_89817617_400000_CN_89818719_400000/LConn2
  DV_Melina___Divača_CN_96747435_400000_CN_89817617_400000/RConn3 -- T_89817617_400000_TS_Melina/LConn3 -- DV_Tumbri___Melina_CN_89817617_400000_CN_89818719_400000/LConn3 -- bus83/LConn1
  T_89818719_400000_TS_Tumbri/LConn1 -- DV_Tumbri___Melina_CN_89817617_400000_CN_89818719_400000/RConn1
  T_89818719_400000_TS_Tumbri/LConn2 -- DV_Tumbri___Melina_CN_89817617_400000_CN_89818719_400000/RConn2
  DV_Tumbri___Melina_CN_89817617_400000_CN_89818719_400000/RConn3 -- T_89818719_400000_TS_Tumbri/LConn3 -- bus84/LConn1
  G_119239942_Termoelektrarna_Šoštanj/RConn1 -- 400_kV_RTP_Šoštanj_RTP_Podlog_CN_119244495_400000_CN_119239942_400000/RConn1
  G_119239942_Termoelektrarna_Šoštanj/RConn2 -- 400_kV_RTP_Šoštanj_RTP_Podlog_CN_119244495_400000_CN_119239942_400000/RConn2
  400_kV_RTP_Šoštanj_RTP_Podlog_CN_119244495_400000_CN_119239942_400000/RConn3 -- G_119239942_Termoelektrarna_Šoštanj/RConn3 -- bus85/LConn1
  T_199309340__RTP_Ozbalt/RConn1 -- L_199309340/LConn1
  T_199309340__RTP_Ozbalt/RConn2 -- L_199309340/LConn2
  L_199309340/LConn3 -- T_199309340__RTP_Ozbalt/RConn3 -- bus86/LConn1
  T_171608231__RTP/RConn1 -- L_171608231/LConn1
  T_171608231__RTP/RConn2 -- L_171608231/LConn2
  L_171608231/LConn3 -- T_171608231__RTP/RConn3 -- bus87/LConn1
  T_129377014__HE_Vuhred/RConn1 -- L_129377014/LConn1
  T_129377014__HE_Vuhred/RConn2 -- L_129377014/LConn2
  L_129377014/LConn3 -- T_129377014__HE_Vuhred/RConn3 -- bus88/LConn1
  T_121547295_110000_HE_Mavčiče/RConn1 -- L_121547295/LConn1
  T_121547295_110000_HE_Mavčiče/RConn2 -- L_121547295/LConn2
  L_121547295/LConn3 -- T_121547295_110000_HE_Mavčiče/RConn3 -- bus89/LConn1
  T_306834171__RTP_Labore/RConn1 -- L_306834171/LConn1
  T_306834171__RTP_Labore/RConn2 -- L_306834171/LConn2
  L_306834171/LConn3 -- T_306834171__RTP_Labore/RConn3 -- bus90/LConn1
  T_167068843_220000;110000_RTP_Kleče/RConn1 -- L_167068843/LConn1
  T_167068843_220000;110000_RTP_Kleče/RConn2 -- L_167068843/LConn2
  L_167068843/LConn3 -- T_167068843_220000;110000_RTP_Kleče/RConn3 -- bus91/LConn1
  T_34853414__RTP_Pekre/RConn1 -- L_34853414/LConn1
  T_34853414__RTP_Pekre/RConn2 -- L_34853414/LConn2
  L_34853414/LConn3 -- T_34853414__RTP_Pekre/RConn3 -- bus92/LConn1
  T_171257375__RTP_Slovenska_BIstrica/RConn1 -- L_171257375/LConn1
  T_171257375__RTP_Slovenska_BIstrica/RConn2 -- L_171257375/LConn2
  L_171257375/LConn3 -- T_171257375__RTP_Slovenska_BIstrica/RConn3 -- bus93/LConn1
  T_171247394__HE_Mariborski_otok/RConn1 -- L_171247394/LConn1
  T_171247394__HE_Mariborski_otok/RConn2 -- L_171247394/LConn2
  L_171247394/LConn3 -- T_171247394__HE_Mariborski_otok/RConn3 -- bus94/LConn1
  T_171242382__RTP_Koroška_vrata/RConn1 -- L_171242382/LConn1
  T_171242382__RTP_Koroška_vrata/RConn2 -- L_171242382/LConn2
  L_171242382/LConn3 -- T_171242382__RTP_Koroška_vrata/RConn3 -- bus95/LConn1
  T_170856590__RTP_Dobrava/RConn1 -- L_170856590/LConn1
  T_170856590__RTP_Dobrava/RConn2 -- L_170856590/LConn2
  L_170856590/LConn3 -- T_170856590__RTP_Dobrava/RConn3 -- bus96/LConn1
  T_280821359__/RConn1 -- L_280821359/LConn1
  T_280821359__/RConn2 -- L_280821359/LConn2
  L_280821359/LConn3 -- T_280821359__/RConn3 -- bus97/LConn1
  T_171277752__RTP_Slovenske_Konjice/RConn1 -- L_171277752/LConn1
  T_171277752__RTP_Slovenske_Konjice/RConn2 -- L_171277752/LConn2
  L_171277752/LConn3 -- T_171277752__RTP_Slovenske_Konjice/RConn3 -- bus98/LConn1
  T_171047486__RTP_Kidričevo/RConn1 -- L_171047486/LConn1
  T_171047486__RTP_Kidričevo/RConn2 -- L_171047486/LConn2
  L_171047486/LConn3 -- T_171047486__RTP_Kidričevo/RConn3 -- bus99/LConn1
  T_113568896__RTP_Cirkovce/RConn1 -- L_113568896/LConn1
  T_113568896__RTP_Cirkovce/RConn2 -- L_113568896/LConn2
  L_113568896/LConn3 -- T_113568896__RTP_Cirkovce/RConn3 -- bus100/LConn1
  T_171127243__RTP_Ptuj/RConn1 -- L_171127243/LConn1
  T_171127243__RTP_Ptuj/RConn2 -- L_171127243/LConn2
  L_171127243/LConn3 -- T_171127243__RTP_Ptuj/RConn3 -- bus101/LConn1
  T_198587974__RTP/RConn1 -- L_198587974/LConn1
  T_198587974__RTP/RConn2 -- L_198587974/LConn2
  L_198587974/LConn3 -- T_198587974__RTP/RConn3 -- bus102/LConn1
  T_199456336__RTP_Bršljin/RConn1 -- L_199456336/LConn1
  T_199456336__RTP_Bršljin/RConn2 -- L_199456336/LConn2
  L_199456336/LConn3 -- T_199456336__RTP_Bršljin/RConn3 -- bus103/LConn1
  T_198740080_110000_RP_Hudo/RConn1 -- L_198740080/LConn1
  T_198740080_110000_RP_Hudo/RConn2 -- L_198740080/LConn2
  L_198740080/LConn3 -- T_198740080_110000_RP_Hudo/RConn3 -- bus104/LConn1
  T_199456340_110000_RTP_Grosuplje/RConn1 -- L_199456340/LConn1
  T_199456340_110000_RTP_Grosuplje/RConn2 -- L_199456340/LConn2
  L_199456340/LConn3 -- T_199456340_110000_RTP_Grosuplje/RConn3 -- bus105/LConn1
  T_199456341__RTP_Kamnik/RConn1 -- L_199456341/LConn1
  T_199456341__RTP_Kamnik/RConn2 -- L_199456341/LConn2
  L_199456341/LConn3 -- T_199456341__RTP_Kamnik/RConn3 -- bus106/LConn1
  T_198965564__RTP_Domžale/RConn1 -- L_198965564/LConn1
  T_198965564__RTP_Domžale/RConn2 -- L_198965564/LConn2
  L_198965564/LConn3 -- T_198965564__RTP_Domžale/RConn3 -- bus107/LConn1
  T_199456345__RTP_Potoška_vas/RConn1 -- L_199456345/LConn1
  T_199456345__RTP_Potoška_vas/RConn2 -- L_199456345/LConn2
  L_199456345/LConn3 -- T_199456345__RTP_Potoška_vas/RConn3 -- bus108/LConn1
  T_286599451__RTP_Trbovlje/RConn1 -- L_286599451/LConn1
  T_286599451__RTP_Trbovlje/RConn2 -- L_286599451/LConn2
  L_286599451/LConn3 -- T_286599451__RTP_Trbovlje/RConn3 -- bus109/LConn1
  T_199456347__RTP_Vič/RConn1 -- L_199456347/LConn1
  T_199456347__RTP_Vič/RConn2 -- L_199456347/LConn2
  L_199456347/LConn3 -- T_199456347__RTP_Vič/RConn3 -- bus110/LConn1
  T_199456348__RTP_Šiška/RConn1 -- L_199456348/LConn1
  T_199456348__RTP_Šiška/RConn2 -- L_199456348/LConn2
  L_199456348/LConn3 -- T_199456348__RTP_Šiška/RConn3 -- bus111/LConn1
  T_198740079__/RConn1 -- L_198740079/LConn1
  T_198740079__/RConn2 -- L_198740079/LConn2
  L_198740079/LConn3 -- T_198740079__/RConn3 -- bus112/LConn1
  T_262103381__/RConn1 -- L_262103381/LConn1
  T_262103381__/RConn2 -- L_262103381/LConn2
  L_262103381/LConn3 -- T_262103381__/RConn3 -- bus113/LConn1
  T_306794096_110000_HE_Plave/RConn1 -- L_306794096/LConn1
  T_306794096_110000_HE_Plave/RConn2 -- L_306794096/LConn2
  L_306794096/LConn3 -- T_306794096_110000_HE_Plave/RConn3 -- bus114/LConn1
  T_370156011__RTP_Anhovo/RConn1 -- L_370156011/LConn1
  T_370156011__RTP_Anhovo/RConn2 -- L_370156011/LConn2
  L_370156011/LConn3 -- T_370156011__RTP_Anhovo/RConn3 -- bus115/LConn1
  T_280821361__/RConn1 -- L_280821361/LConn1
  T_280821361__/RConn2 -- L_280821361/LConn2
  L_280821361/LConn3 -- T_280821361__/RConn3 -- bus116/LConn1
  T_280821367__/RConn1 -- L_280821367/LConn1
  T_280821367__/RConn2 -- L_280821367/LConn2
  L_280821367/LConn3 -- T_280821367__/RConn3 -- bus117/LConn1
  T_199131958__RTP_Logatec/RConn1 -- L_199131958/LConn1
  T_199131958__RTP_Logatec/RConn2 -- L_199131958/LConn2
  L_199131958/LConn3 -- T_199131958__RTP_Logatec/RConn3 -- bus118/LConn1
  T_199131955__RTP_Vrhnika/RConn1 -- L_199131955/LConn1
  T_199131955__RTP_Vrhnika/RConn2 -- L_199131955/LConn2
  L_199131955/LConn3 -- T_199131955__RTP_Vrhnika/RConn3 -- bus119/LConn1
  T_172406389__RTP_Radenci/RConn1 -- L_172406389/LConn1
  T_172406389__RTP_Radenci/RConn2 -- L_172406389/LConn2
  L_172406389/LConn3 -- T_172406389__RTP_Radenci/RConn3 -- bus120/LConn1
  T_172405235__RTP_Murska_Sobota/RConn1 -- L_172405235/LConn1
  T_172405235__RTP_Murska_Sobota/RConn2 -- L_172405235/LConn2
  L_172405235/LConn3 -- T_172405235__RTP_Murska_Sobota/RConn3 -- bus121/LConn1
  T_171229302__RTP_Ljutomer/RConn1 -- L_171229302/LConn1
  T_171229302__RTP_Ljutomer/RConn2 -- L_171229302/LConn2
  L_171229302/LConn3 -- T_171229302__RTP_Ljutomer/RConn3 -- bus122/LConn1
  T_200118427__/RConn1 -- L_200118427/LConn1
  T_200118427__/RConn2 -- L_200118427/LConn2
  L_200118427/LConn3 -- T_200118427__/RConn3 -- bus123/LConn1
  T_171227992__RTP_Ormož/RConn1 -- L_171227992/LConn1
  T_171227992__RTP_Ormož/RConn2 -- L_171227992/LConn2
  L_171227992/LConn3 -- T_171227992__RTP_Ormož/RConn3 -- bus124/LConn1
  T_280821368__/RConn1 -- L_280821368/LConn1
  T_280821368__/RConn2 -- L_280821368/LConn2
  L_280821368/LConn3 -- T_280821368__/RConn3 -- bus125/LConn1
  T_262103358__/RConn1 -- L_262103358/LConn1
  T_262103358__/RConn2 -- L_262103358/LConn2
  L_262103358/LConn3 -- T_262103358__/RConn3 -- bus126/LConn1
  T_159593130__TS_Straža/RConn1 -- L_159593130/LConn1
  T_159593130__TS_Straža/RConn2 -- L_159593130/LConn2
  L_159593130/LConn3 -- T_159593130__TS_Straža/RConn3 -- bus127/LConn1
  T_208625989__/RConn1 -- L_208625989/LConn1
  T_208625989__/RConn2 -- L_208625989/LConn2
  L_208625989/LConn3 -- T_208625989__/RConn3 -- bus128/LConn1
  T_99634141__TS_Ivanec/RConn1 -- L_99634141/LConn1
  T_99634141__TS_Ivanec/RConn2 -- L_99634141/LConn2
  L_99634141/LConn3 -- T_99634141__TS_Ivanec/RConn3 -- bus129/LConn1
  T_306834196__RTP_Škofja_Loka/RConn1 -- L_306834196/LConn1
  T_306834196__RTP_Škofja_Loka/RConn2 -- L_306834196/LConn2
  L_306834196/LConn3 -- T_306834196__RTP_Škofja_Loka/RConn3 -- bus130/LConn1
  T_186330420__RTP_Črnuče/RConn1 -- L_186330420/LConn1
  T_186330420__RTP_Črnuče/RConn2 -- L_186330420/LConn2
  L_186330420/LConn3 -- T_186330420__RTP_Črnuče/RConn3 -- bus131/LConn1
  T_376534710__RTP/RConn1 -- L_376534710/LConn1
  T_376534710__RTP/RConn2 -- L_376534710/LConn2
  L_376534710/LConn3 -- T_376534710__RTP/RConn3 -- bus132/LConn1
  T_132468928_110000_Kraftwerk_Koralpe/RConn1 -- L_132468928/LConn1
  T_132468928_110000_Kraftwerk_Koralpe/RConn2 -- L_132468928/LConn2
  L_132468928/LConn3 -- T_132468928_110000_Kraftwerk_Koralpe/RConn3 -- bus133/LConn1
  T_161693379__RTP/RConn1 -- L_161693379/LConn1
  T_161693379__RTP/RConn2 -- L_161693379/LConn2
  L_161693379/LConn3 -- T_161693379__RTP/RConn3 -- bus134/LConn1
  T_198773972__/RConn1 -- L_198773972/LConn1
  T_198773972__/RConn2 -- L_198773972/LConn2
  L_198773972/LConn3 -- T_198773972__/RConn3 -- bus135/LConn1
  T_128572102__TS_Matulji/RConn1 -- L_128572102/LConn1
  T_128572102__TS_Matulji/RConn2 -- L_128572102/LConn2
  L_128572102/LConn3 -- T_128572102__TS_Matulji/RConn3 -- bus136/LConn1
  T_276296152__Ilirska_Bistrica/RConn1 -- L_276296152/LConn1
  T_276296152__Ilirska_Bistrica/RConn2 -- L_276296152/LConn2
  L_276296152/LConn3 -- T_276296152__Ilirska_Bistrica/RConn3 -- bus137/LConn1
  T_198773974__RTP_Vuzenica/RConn1 -- L_198773974/LConn1
  T_198773974__RTP_Vuzenica/RConn2 -- L_198773974/LConn2
  L_198773974/LConn3 -- T_198773974__RTP_Vuzenica/RConn3 -- bus138/LConn1
  T_306834179__RTP_Primskovo/RConn1 -- L_306834179/LConn1
  T_306834179__RTP_Primskovo/RConn2 -- L_306834179/LConn2
  L_306834179/LConn3 -- T_306834179__RTP_Primskovo/RConn3 -- bus139/LConn1
  T_242310951_110000_RTP_Postojna/RConn1 -- L_242310951/LConn1
  T_242310951_110000_RTP_Postojna/RConn2 -- L_242310951/LConn2
  L_242310951/LConn3 -- T_242310951_110000_RTP_Postojna/RConn3 -- bus140/LConn1
  T_199389074_110000_RTP_Pivka/RConn1 -- L_199389074/LConn1
  T_199389074_110000_RTP_Pivka/RConn2 -- L_199389074/LConn2
  L_199389074/LConn3 -- T_199389074_110000_RTP_Pivka/RConn3 -- bus141/LConn1
  T_199131954__RTP_Koper/RConn1 -- L_199131954/LConn1
  T_199131954__RTP_Koper/RConn2 -- L_199131954/LConn2
  L_199131954/LConn3 -- T_199131954__RTP_Koper/RConn3 -- bus142/LConn1
  T_123454320__TS_Buje/RConn1 -- L_123454320/LConn1
  T_123454320__TS_Buje/RConn2 -- L_123454320/LConn2
  L_123454320/LConn3 -- T_123454320__TS_Buje/RConn3 -- bus143/LConn1
  T_208270146__RTP/RConn1 -- L_208270146/LConn1
  T_208270146__RTP/RConn2 -- L_208270146/LConn2
  L_208270146/LConn3 -- T_208270146__RTP/RConn3 -- bus144/LConn1
  T_306692456_110000_RTP_Vrtojba/RConn1 -- L_306692456/LConn1
  T_306692456_110000_RTP_Vrtojba/RConn2 -- L_306692456/LConn2
  L_306692456/LConn3 -- T_306692456_110000_RTP_Vrtojba/RConn3 -- bus145/LConn1
  T_306692448_110000_RTP_Nova_Gorica/RConn1 -- L_306692448/LConn1
  T_306692448_110000_RTP_Nova_Gorica/RConn2 -- L_306692448/LConn2
  L_306692448/LConn3 -- T_306692448_110000_RTP_Nova_Gorica/RConn3 -- bus146/LConn1
  T_369889747_110000_RTP_Tolmin/RConn1 -- L_369889747/LConn1
  T_369889747_110000_RTP_Tolmin/RConn2 -- L_369889747/LConn2
  L_369889747/LConn3 -- T_369889747_110000_RTP_Tolmin/RConn3 -- bus147/LConn1
  T_171246987__RTP_Lenart/RConn1 -- L_171246987/LConn1
  T_171246987__RTP_Lenart/RConn2 -- L_171246987/LConn2
  L_171246987/LConn3 -- T_171246987__RTP_Lenart/RConn3 -- bus148/LConn1
  T_171242383__RTP_Melje/RConn1 -- L_171242383/LConn1
  T_171242383__RTP_Melje/RConn2 -- L_171242383/LConn2
  L_171242383/LConn3 -- T_171242383__RTP_Melje/RConn3 -- bus149/LConn1
  T_138362817__RTP_Polje/RConn1 -- L_138362817/LConn1
  T_138362817__RTP_Polje/RConn2 -- L_138362817/LConn2
  L_138362817/LConn3 -- T_138362817__RTP_Polje/RConn3 -- bus150/LConn1
  T_105894370__RTP_Krško/RConn1 -- L_105894370/LConn1
  T_105894370__RTP_Krško/RConn2 -- L_105894370/LConn2
  L_105894370/LConn3 -- T_105894370__RTP_Krško/RConn3 -- bus151/LConn1
  T_89817617_400000_TS_Melina/RConn1 -- L_89817617/LConn1
  T_89817617_400000_TS_Melina/RConn2 -- L_89817617/LConn2
  L_89817617/LConn3 -- T_89817617_400000_TS_Melina/RConn3 -- bus152/LConn1
  T_89818719_400000_TS_Tumbri/RConn1 -- L_89818719/LConn1
  T_89818719_400000_TS_Tumbri/RConn2 -- L_89818719/LConn2
  L_89818719/LConn3 -- T_89818719_400000_TS_Tumbri/RConn3 -- bus153/LConn1
